simulink model "Taxi_park_hcs"  (R2022a)
settings: Solver=VariableStepAuto  StartTime=0.0  StopTime=10.0  RelTol=1e-3
settings Model: Creator=ayj  LastModifiedBy=ayj

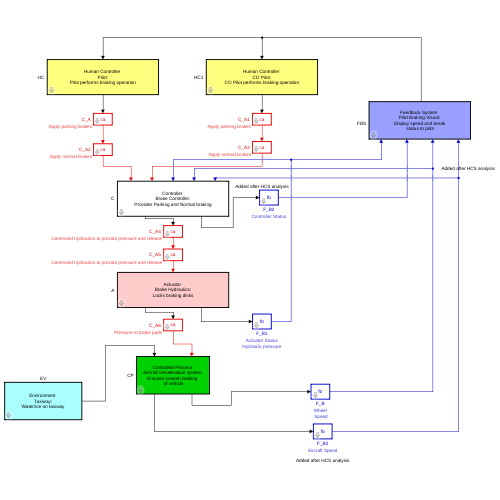
[thumbnail: Simulink's stored preview of the top-level diagram]
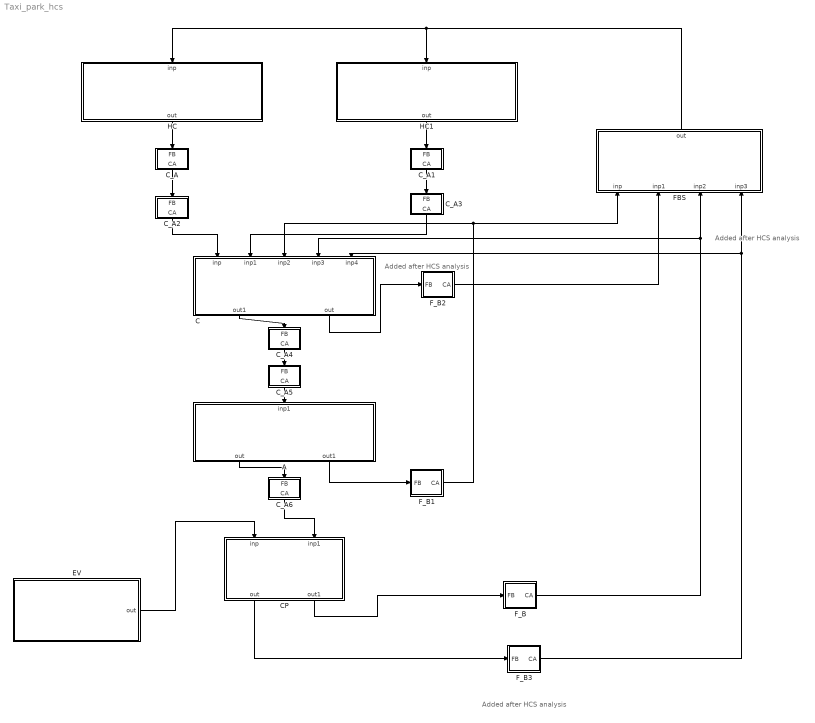
== system Taxi_park_hcs ==
  note: Added after HCS analysis
  note: Added after HCS analysis
  note: Added after HCS analysis
  " FBS" : Subsystem  TreatAsAtomicUnit=on  mask(feedback_system){NAMEFORBLOCK=Pilot Braking Visual, DES=Display speed and break\n status to pilot}
      mask prompts: NAMEFORBLOCK "Provide a name"; DES "Provide a description of feedback system"
      mask help: Say what this feedback system does
      mask init:
      | set_param(gcb,'LinkStatus', 'none');
      settings: RTWFcnNameOpts=Use subsystem name  RTWFileNameOpts=Use function name
      mask DialogControl Control2 Prompt: ADD Input
      mask DialogControl Control2 Callback:
      | h = add_block('simulink/Sources/In1', [gcb '/inp'], 'MakeNameUnique', 'on');
      | hg = add_block('simulink/Sinks/Terminator', [gcb '/term'], 'MakeNameUnique', 'on');
      | hname = get_param(h,'PortHandles');
      | hgname = get_param(hg,'PortHandles');
      | add_line(gcb, hname.Outport(1), hgname.Inport(1));
      mask DialogControl Control3 Prompt: ADD Output
      mask DialogControl Control3 Callback:
      | h = add_block('simulink/Sinks/Out1', [gcb '/out'], 'MakeNameUnique', 'on');
      | hg = add_block('simulink/Sources/Ground', [gcb '/gnd'], 'MakeNameUnique', 'on');
      | hname = get_param(h,'PortHandles');
      | hgname = get_param(hg,'PortHandles');
      | add_line(gcb, hgname.Outport(1), hname.Inport(1));
      mask DialogControl Control4 Prompt: REM Input
      mask DialogControl Control4 Callback:
      | a=find_system(gcb,'SearchDepth',2,'LookUnderMasks','all','BlockType','Inport');
      | if ~isempty(a)
      | b=get_param(a{1},'PortConnectivity');
      | delete_block(a{1});
      | delete_block(b.DstBlock);
      | delete_line(find_system(gcb, 'SearchDepth',2,'LookUnderMasks','all','FindAll', 'on', 'Type', 'line', 'Connected', 'off'))
      | end
      mask DialogControl Control5 Prompt: REM Output
      mask DialogControl Control5 Callback:
      | a=find_system(gcb,'SearchDepth',2,'LookUnderMasks','all','BlockType','Outport');
      | if ~isempty(a)
      | b=get_param(a{1},'PortConnectivity');
      | delete_block(a{1});
      | delete_block(b.SrcBlock);
      | delete_line(find_system(gcb, 'SearchDepth',2,'LookUnderMasks','all','FindAll', 'on', 'Type', 'line', 'Connected', 'off'))
      | end
      mask Display: disp(['Feedback System \n' NAMEFORBLOCK ':\n' DES])
  A : Subsystem  TreatAsAtomicUnit=on  mask(actuator){NAMEFORBLOCK=Brake Hydraulics, DES=Locks braking disks}
      mask prompts: NAMEFORBLOCK "Provide a name for Block"; DES "Provide a description of Responsibility"
      mask help: Say what this actuator does
      mask init:
      | set_param(gcb,'LinkStatus', 'none');
      settings: RTWFcnNameOpts=Use subsystem name  RTWFileNameOpts=Use function name
      mask DialogControl Control2 Prompt: ADD Input
      mask DialogControl Control2 Callback:
      | h = add_block('simulink/Sources/In1', [gcb '/inp'], 'MakeNameUnique', 'on');
      | hg = add_block('simulink/Sinks/Terminator', [gcb '/term'], 'MakeNameUnique', 'on');
      | hname = get_param(h,'PortHandles');
      | hgname = get_param(hg,'PortHandles');
      | add_line(gcb, hname.Outport(1), hgname.Inport(1));
      mask DialogControl Control3 Prompt: ADD Output
      mask DialogControl Control3 Callback:
      | h = add_block('simulink/Sinks/Out1', [gcb '/out'], 'MakeNameUnique', 'on');
      | hg = add_block('simulink/Sources/Ground', [gcb '/gnd'], 'MakeNameUnique', 'on');
      | hname = get_param(h,'PortHandles');
      | hgname = get_param(hg,'PortHandles');
      | add_line(gcb, hgname.Outport(1), hname.Inport(1));
      mask DialogControl Control4 Prompt: REM Input
      mask DialogControl Control4 Callback:
      | a=find_system(gcb,'SearchDepth',2,'LookUnderMasks','all','BlockType','Inport');
      | if ~isempty(a)
      | b=get_param(a{1},'PortConnectivity');
      | delete_block(a{1});
      | delete_block(b.DstBlock);
      | delete_line(find_system(gcb, 'SearchDepth',2,'LookUnderMasks','all','FindAll', 'on', 'Type', 'line', 'Connected', 'off'))
      | end
      mask DialogControl Control5 Prompt: REM Output
      mask DialogControl Control5 Callback:
      | a=find_system(gcb,'SearchDepth',2,'LookUnderMasks','all','BlockType','Outport');
      | if ~isempty(a)
      | b=get_param(a{1},'PortConnectivity');
      | delete_block(a{1});
      | delete_block(b.SrcBlock);
      | delete_line(find_system(gcb, 'SearchDepth',2,'LookUnderMasks','all','FindAll', 'on', 'Type', 'line', 'Connected', 'off'))
      | end
      mask Display: disp(['Actuator \n' NAMEFORBLOCK ':\n' DES])
  C : Subsystem  TreatAsAtomicUnit=on  mask(controller){NAMEFORBLOCK=Brake Controller, DES=Provides Parking and Normal braking}
      mask prompts: NAMEFORBLOCK "Provide a name for Block"; DES "Provide a description of Responsibility"
      mask help: Say what this controller does
      mask init:
      | set_param(gcb,'LinkStatus', 'none');
      settings: RTWFcnNameOpts=Use subsystem name  RTWFileNameOpts=Use function name
      mask DialogControl Control2 Prompt: ADD Input
      mask DialogControl Control2 Callback:
      | h = add_block('simulink/Sources/In1', [gcb '/inp'], 'MakeNameUnique', 'on');
      | hg = add_block('simulink/Sinks/Terminator', [gcb '/term'], 'MakeNameUnique', 'on');
      | hname = get_param(h,'PortHandles');
      | hgname = get_param(hg,'PortHandles');
      | add_line(gcb, hname.Outport(1), hgname.Inport(1));
      mask DialogControl Control3 Prompt: ADD Output
      mask DialogControl Control3 Callback:
      | h = add_block('simulink/Sinks/Out1', [gcb '/out'], 'MakeNameUnique', 'on');
      | hg = add_block('simulink/Sources/Ground', [gcb '/gnd'], 'MakeNameUnique', 'on');
      | hname = get_param(h,'PortHandles');
      | hgname = get_param(hg,'PortHandles');
      | add_line(gcb, hgname.Outport(1), hname.Inport(1));
      mask DialogControl Control4 Prompt: REM Input
      mask DialogControl Control4 Callback:
      | a=find_system(gcb,'SearchDepth',2,'LookUnderMasks','all','BlockType','Inport');
      | if ~isempty(a)
      | b=get_param(a{1},'PortConnectivity');
      | delete_block(a{1});
      | delete_block(b.DstBlock);
      | delete_line(find_system(gcb, 'SearchDepth',2,'LookUnderMasks','all','FindAll', 'on', 'Type', 'line', 'Connected', 'off'))
      | end
      mask DialogControl Control5 Prompt: REM Output
      mask DialogControl Control5 Callback:
      | a=find_system(gcb,'SearchDepth',2,'LookUnderMasks','all','BlockType','Outport');
      | if ~isempty(a)
      | b=get_param(a{1},'PortConnectivity');
      | delete_block(a{1});
      | delete_block(b.SrcBlock);
      | delete_line(find_system(gcb, 'SearchDepth',2,'LookUnderMasks','all','FindAll', 'on', 'Type', 'line', 'Connected', 'off'))
      | end
      mask Display: disp(['Controller \n' NAMEFORBLOCK ':\n' DES])
  CP : Subsystem  TreatAsAtomicUnit=on  mask(controlled_process){NAMEFORBLOCK=Aircraft Deceleration system, DES=Ensures smooth braking \n of vehicle}
      mask prompts: NAMEFORBLOCK "Provide a name for Block"; DES "Provide a description of Responsibility"
      mask help: Say what this controlled process does
      settings: RTWFcnNameOpts=Use subsystem name  RTWFileNameOpts=Use function name
      mask DialogControl Control2 Prompt: ADD Input
      mask DialogControl Control2 Callback:
      | set_param(gcb,'LinkStatus', 'none');
      | h = add_block('simulink/Sources/In1', [gcb '/inp'], 'MakeNameUnique', 'on');
      | hg = add_block('simulink/Sinks/Terminator', [gcb '/term'], 'MakeNameUnique', 'on');
      | hname = get_param(h,'PortHandles');
      | hgname = get_param(hg,'PortHandles');
      | add_line(gcb, hname.Outport(1), hgname.Inport(1));
      mask DialogControl Control3 Prompt: ADD Output
      mask DialogControl Control3 Callback:
      | set_param(gcb,'LinkStatus', 'none');
      | h = add_block('simulink/Sinks/Out1', [gcb '/out'], 'MakeNameUnique', 'on');
      | hg = add_block('simulink/Sources/Ground', [gcb '/gnd'], 'MakeNameUnique', 'on');
      | hname = get_param(h,'PortHandles');
      | hgname = get_param(hg,'PortHandles');
      | add_line(gcb, hgname.Outport(1), hname.Inport(1));
      mask DialogControl Control4 Prompt: REM Input
      mask DialogControl Control4 Callback:
      | set_param(gcb,'LinkStatus', 'none');
      | a=find_system(gcb,'SearchDepth',2,'LookUnderMasks','all','BlockType','Inport');
      | if ~isempty(a)
      | b=get_param(a{1},'PortConnectivity');
      | delete_block(a{1});
      | delete_block(b.DstBlock);
      | delete_line(find_system(gcb, 'SearchDepth',2,'LookUnderMasks','all','FindAll', 'on', 'Type', 'line', 'Connected', 'off'))
      | end
      mask DialogControl Control5 Prompt: REM Output
      mask DialogControl Control5 Callback:
      | set_param(gcb,'LinkStatus', 'none');
      | a=find_system(gcb,'SearchDepth',2,'LookUnderMasks','all','BlockType','Outport');
      | if ~isempty(a)
      | b=get_param(a{1},'PortConnectivity');
      | delete_block(a{1});
      | delete_block(b.SrcBlock);
      | delete_line(find_system(gcb, 'SearchDepth',2,'LookUnderMasks','all','FindAll', 'on', 'Type', 'line', 'Connected', 'off'))
      | end
      mask Display: disp(['Controlled Process \n' NAMEFORBLOCK ':\n' DES])
  C_A : Subsystem  TreatAsAtomicUnit=on  mask(control_action){DES=Apply parking brakes, UCA1=[#H5_1] Not providing at parking zone, UCA2=[#H4] Providing when taxing out, UCA3=[#H4] Providing early before aircraft has stopped, UCA4=}
      mask prompts: DES "Provide a description of Control Action"; UCA1 "Not providing causes hazard [link Hazard]"; UCA2 "Providing causes hazard [link Hazard]"; UCA3 "Too early, too late, out of order [link Hazard]"; UCA4 "Stopped too soon, applied too long [link Hazard]"
      mask help:
      | <Source> <Type> <Control Action> <Context> <Link to Hazards>
      | Source = System Above, Type = {provided, not provided ..], Control Action = command
      | from the description, Context = While/When .. Always link to a hazard
      mask init:
      | set_param(gcb,'LinkStatus', 'none');
      settings: AttributesFormatString=%<DES>  RTWFcnNameOpts=Use subsystem name  RTWFileNameOpts=Use function name
      mask Display: disp('ca')
  C_A1 : Subsystem  TreatAsAtomicUnit=on  mask(control_action){DES=Apply parking brakes, UCA1=[#H5_1] Not providing at parking zone, UCA2=[#H4] Providing when taxing out, UCA3=[#H4] Providing early before aircraft has stopped, UCA4=}
      mask prompts: DES "Provide a description of Control Action"; UCA1 "Not providing causes hazard [link Hazard]"; UCA2 "Providing causes hazard [link Hazard]"; UCA3 "Too early, too late, out of order [link Hazard]"; UCA4 "Stopped too soon, applied too long [link Hazard]"
      mask help:
      | <Source> <Type> <Control Action> <Context> <Link to Hazards>
      | Source = System Above, Type = {provided, not provided ..], Control Action = command
      | from the description, Context = While/When .. Always link to a hazard
      mask init:
      | set_param(gcb,'LinkStatus', 'none');
      settings: AttributesFormatString=%<DES>  RTWFcnNameOpts=Use subsystem name  RTWFileNameOpts=Use function name
      mask Display: disp('ca')
  C_A2 : Subsystem  TreatAsAtomicUnit=on  mask(control_action){DES=Apply normal brakes, UCA1=[#H5, #H6] Not applying brakes when instructed/needed, UCA2=[#H6] Providing without informing, UCA3=[#H4, #H7] erractic application of brakes, UCA4=[#H4, #H6] Release break before speed 0}
      mask prompts: DES "Provide a description of Control Action"; UCA1 "Not providing causes hazard [link Hazard]"; UCA2 "Providing causes hazard [link Hazard]"; UCA3 "Too early, too late, out of order [link Hazard]"; UCA4 "Stopped too soon, applied too long [link Hazard]"
      mask help:
      | <Source> <Type> <Control Action> <Context> <Link to Hazards>
      | Source = System Above, Type = {provided, not provided ..], Control Action = command
      | from the description, Context = While/When .. Always link to a hazard
      mask init:
      | set_param(gcb,'LinkStatus', 'none');
      settings: AttributesFormatString=%<DES>  RTWFcnNameOpts=Use subsystem name  RTWFileNameOpts=Use function name
      mask Display: disp('ca')
  C_A3 : Subsystem  TreatAsAtomicUnit=on  mask(control_action){DES=Apply normal brakes, UCA1=[#H5, #H6] Not applying brakes when instructed/needed, UCA2=[#H6] Providing without informing, UCA3=[#H4, #H7] erractic application of brakes, UCA4=[#H4, #H6] Release break before speed 0}
      mask prompts: DES "Provide a description of Control Action"; UCA1 "Not providing causes hazard [link Hazard]"; UCA2 "Providing causes hazard [link Hazard]"; UCA3 "Too early, too late, out of order [link Hazard]"; UCA4 "Stopped too soon, applied too long [link Hazard]"
      mask help:
      | <Source> <Type> <Control Action> <Context> <Link to Hazards>
      | Source = System Above, Type = {provided, not provided ..], Control Action = command
      | from the description, Context = While/When .. Always link to a hazard
      mask init:
      | set_param(gcb,'LinkStatus', 'none');
      settings: AttributesFormatString=%<DES>  RTWFcnNameOpts=Use subsystem name  RTWFileNameOpts=Use function name
      mask Display: disp('ca')
  C_A4 : Subsystem  TreatAsAtomicUnit=on  mask(control_action){DES=Command hydraulics to provide pressure and release, UCA1=[#H5, #H6] Not providing when demanded by pilot, UCA2=[#H5, #H6] Providing when pilot does not demand, UCA3=[#H5, #H6] Delayed brake action on command, UCA4=[#H5, #H6] Stopping brake pressure even under demand}
      mask prompts: DES "Provide a description of Control Action"; UCA1 "Not providing causes hazard [link Hazard]"; UCA2 "Providing causes hazard [link Hazard]"; UCA3 "Too early, too late, out of order [link Hazard]"; UCA4 "Stopped too soon, applied too long [link Hazard]"
      mask help:
      | <Source> <Type> <Control Action> <Context> <Link to Hazards>
      | Source = System Above, Type = {provided, not provided ..], Control Action = command
      | from the description, Context = While/When .. Always link to a hazard
      mask init:
      | set_param(gcb,'LinkStatus', 'none');
      settings: AttributesFormatString=%<DES>  RTWFcnNameOpts=Use subsystem name  RTWFileNameOpts=Use function name
      mask Display: disp('ca')
  C_A5 : Subsystem  TreatAsAtomicUnit=on  mask(control_action){DES=Command hydraulics to provide pressure and release, UCA1=, UCA2=[#H5, #H6] Providing unequal pressure to wheels, UCA3=[#H5, #H6] Either of the brakes are not in sync, UCA4=}
      mask prompts: DES "Provide a description of Control Action"; UCA1 "Not providing causes hazard [link Hazard]"; UCA2 "Providing causes hazard [link Hazard]"; UCA3 "Too early, too late, out of order [link Hazard]"; UCA4 "Stopped too soon, applied too long [link Hazard]"
      mask help:
      | <Source> <Type> <Control Action> <Context> <Link to Hazards>
      | Source = System Above, Type = {provided, not provided ..], Control Action = command
      | from the description, Context = While/When .. Always link to a hazard
      mask init:
      | set_param(gcb,'LinkStatus', 'none');
      settings: AttributesFormatString=%<DES>  RTWFcnNameOpts=Use subsystem name  RTWFileNameOpts=Use function name
      mask Display: disp('ca')
  C_A6 : Subsystem  TreatAsAtomicUnit=on  mask(control_action){DES=Pressure to brake pads, UCA1=[#H5, #H6] Not providing when demanded, UCA2=[#H5, #H6] Providing when not demanded, UCA3=[#H5, #H6] Providing pressure too late, UCA4=[#H5, #H6] Not releasing brake / Releasing too soon}
      mask prompts: DES "Provide a description of Control Action"; UCA1 "Not providing causes hazard [link Hazard]"; UCA2 "Providing causes hazard [link Hazard]"; UCA3 "Too early, too late, out of order [link Hazard]"; UCA4 "Stopped too soon, applied too long [link Hazard]"
      mask help:
      | <Source> <Type> <Control Action> <Context> <Link to Hazards>
      | Source = System Above, Type = {provided, not provided ..], Control Action = command
      | from the description, Context = While/When .. Always link to a hazard
      mask init:
      | set_param(gcb,'LinkStatus', 'none');
      settings: AttributesFormatString=%<DES>  RTWFcnNameOpts=Use subsystem name  RTWFileNameOpts=Use function name
      mask Display: disp('ca')
  EV : Subsystem  TreatAsAtomicUnit=on  mask(environment){NAMEFORBLOCK=Taxiway, DES=Water/ice on taxiway}
      mask prompts: NAMEFORBLOCK "Provide a name for Block"; DES "Provide a description of Interaction"
      mask help: Say how this environment interacts with the system
      mask init:
      | set_param(gcb,'LinkStatus', 'none');
      settings: RTWFcnNameOpts=Use subsystem name  RTWFileNameOpts=Use function name
      mask DialogControl Control2 Prompt: ADD Input
      mask DialogControl Control2 Callback:
      | h = add_block('simulink/Sources/In1', [gcb '/inp'], 'MakeNameUnique', 'on');
      | hg = add_block('simulink/Sinks/Terminator', [gcb '/term'], 'MakeNameUnique', 'on');
      | hname = get_param(h,'PortHandles');
      | hgname = get_param(hg,'PortHandles');
      | add_line(gcb, hname.Outport(1), hgname.Inport(1));
      mask DialogControl Control3 Prompt: ADD Output
      mask DialogControl Control3 Callback:
      | h = add_block('simulink/Sinks/Out1', [gcb '/out'], 'MakeNameUnique', 'on');
      | hg = add_block('simulink/Sources/Ground', [gcb '/gnd'], 'MakeNameUnique', 'on');
      | hname = get_param(h,'PortHandles');
      | hgname = get_param(hg,'PortHandles');
      | add_line(gcb, hgname.Outport(1), hname.Inport(1));
      mask DialogControl Control4 Prompt: REM Input
      mask DialogControl Control4 Callback:
      | a=find_system(gcb,'SearchDepth',2,'LookUnderMasks','all','BlockType','Inport');
      | if ~isempty(a)
      | b=get_param(a{1},'PortConnectivity');
      | delete_block(a{1});
      | delete_block(b.DstBlock);
      | delete_line(find_system(gcb, 'SearchDepth',2,'LookUnderMasks','all','FindAll', 'on', 'Type', 'line', 'Connected', 'off'))
      | end
      mask DialogControl Control5 Prompt: REM Output
      mask DialogControl Control5 Callback:
      | a=find_system(gcb,'SearchDepth',2,'LookUnderMasks','all','BlockType','Outport');
      | if ~isempty(a)
      | b=get_param(a{1},'PortConnectivity');
      | delete_block(a{1});
      | delete_block(b.SrcBlock);
      | delete_line(find_system(gcb, 'SearchDepth',2,'LookUnderMasks','all','FindAll', 'on', 'Type', 'line', 'Connected', 'off'))
      | end
      mask Display: disp(['Environment \n' NAMEFORBLOCK ':\n' DES])
  F_B : Subsystem  TreatAsAtomicUnit=on  mask(feedback){DES=Wheel\n Speed}
      mask prompts: DES "Provide a description"
      mask help: Say what this feeds back from the system
      mask init:
      | set_param(gcb,'LinkStatus', 'none');
      settings: AttributesFormatString=%<DES>  RTWFcnNameOpts=Use subsystem name  RTWFileNameOpts=Use function name
      mask Display: disp('fb')
  F_B1 : Subsystem  TreatAsAtomicUnit=on  mask(feedback){DES=Actuator Status\nHydraulic pressure}
      mask prompts: DES "Provide a description"
      mask help: Say what this feeds back from the system
      mask init:
      | set_param(gcb,'LinkStatus', 'none');
      settings: AttributesFormatString=%<DES>  RTWFcnNameOpts=Use subsystem name  RTWFileNameOpts=Use function name
      mask Display: disp('fb')
  F_B2 : Subsystem  TreatAsAtomicUnit=on  mask(feedback){DES=Controller Status}
      mask prompts: DES "Provide a description"
      mask help: Say what this feeds back from the system
      mask init:
      | set_param(gcb,'LinkStatus', 'none');
      settings: AttributesFormatString=%<DES>  RTWFcnNameOpts=Use subsystem name  RTWFileNameOpts=Use function name
      mask Display: disp('fb')
  F_B3 : Subsystem  TreatAsAtomicUnit=on  mask(feedback){DES=Aircraft Speed}
      mask prompts: DES "Provide a description"
      mask help: Say what this feeds back from the system
      mask init:
      | set_param(gcb,'LinkStatus', 'none');
      settings: AttributesFormatString=%<DES>  RTWFcnNameOpts=Use subsystem name  RTWFileNameOpts=Use function name
      mask Display: disp('fb')
  HC : Subsystem  TreatAsAtomicUnit=on  mask(human_controller){NAMEFORBLOCK=Pilot, DES=Pilot performs braking operation}
      mask prompts: NAMEFORBLOCK "Provide a name for Block"; DES "Provide a description of Responsibility"
      mask help: Say what this human controller does
      mask init:
      | set_param(gcb,'LinkStatus','none')
      settings: RTWFcnNameOpts=Use subsystem name  RTWFileNameOpts=Use function name
      mask DialogControl Control2 Prompt: ADD Input
      mask DialogControl Control2 Callback:
      | h = add_block('simulink/Sources/In1', [gcb '/inp'], 'MakeNameUnique', 'on');
      | hg = add_block('simulink/Sinks/Terminator', [gcb '/term'], 'MakeNameUnique', 'on');
      | hname = get_param(h,'PortHandles');
      | hgname = get_param(hg,'PortHandles');
      | add_line(gcb, hname.Outport(1), hgname.Inport(1));
      mask DialogControl Control3 Prompt: ADD Output
      mask DialogControl Control3 Callback:
      | h = add_block('simulink/Sinks/Out1', [gcb '/out'], 'MakeNameUnique', 'on');
      | hg = add_block('simulink/Sources/Ground', [gcb '/gnd'], 'MakeNameUnique', 'on');
      | hname = get_param(h,'PortHandles');
      | hgname = get_param(hg,'PortHandles');
      | add_line(gcb, hgname.Outport(1), hname.Inport(1));
      mask DialogControl Control4 Prompt: REM Input
      mask DialogControl Control4 Callback:
      | a=find_system(gcb,'SearchDepth',2,'LookUnderMasks','all','BlockType','Inport');
      | if ~isempty(a)
      | b=get_param(a{1},'PortConnectivity');
      | delete_block(a{1});
      | delete_block(b.DstBlock);
      | delete_line(find_system(gcb, 'SearchDepth',2,'LookUnderMasks','all','FindAll', 'on', 'Type', 'line', 'Connected', 'off'))
      | end
      mask DialogControl Control5 Prompt: REM Output
      mask DialogControl Control5 Callback:
      | a=find_system(gcb,'SearchDepth',2,'LookUnderMasks','all','BlockType','Outport');
      | if ~isempty(a)
      | b=get_param(a{1},'PortConnectivity');
      | delete_block(a{1});
      | delete_block(b.SrcBlock);
      | delete_line(find_system(gcb, 'SearchDepth',2,'LookUnderMasks','all','FindAll', 'on', 'Type', 'line', 'Connected', 'off'))
      | end
      mask Display: disp(['Human Controller \n' NAMEFORBLOCK ':\n' DES])
  HC1 : Subsystem  TreatAsAtomicUnit=on  mask(human_controller){NAMEFORBLOCK=CO Pilot, DES=CO Pilot performs braking operation}
      mask prompts: NAMEFORBLOCK "Provide a name for Block"; DES "Provide a description of Responsibility"
      mask help: Say what this human controller does
      mask init:
      | set_param(gcb,'LinkStatus','none')
      settings: RTWFcnNameOpts=Use subsystem name  RTWFileNameOpts=Use function name
      mask DialogControl Control2 Prompt: ADD Input
      mask DialogControl Control2 Callback:
      | h = add_block('simulink/Sources/In1', [gcb '/inp'], 'MakeNameUnique', 'on');
      | hg = add_block('simulink/Sinks/Terminator', [gcb '/term'], 'MakeNameUnique', 'on');
      | hname = get_param(h,'PortHandles');
      | hgname = get_param(hg,'PortHandles');
      | add_line(gcb, hname.Outport(1), hgname.Inport(1));
      mask DialogControl Control3 Prompt: ADD Output
      mask DialogControl Control3 Callback:
      | h = add_block('simulink/Sinks/Out1', [gcb '/out'], 'MakeNameUnique', 'on');
      | hg = add_block('simulink/Sources/Ground', [gcb '/gnd'], 'MakeNameUnique', 'on');
      | hname = get_param(h,'PortHandles');
      | hgname = get_param(hg,'PortHandles');
      | add_line(gcb, hgname.Outport(1), hname.Inport(1));
      mask DialogControl Control4 Prompt: REM Input
      mask DialogControl Control4 Callback:
      | a=find_system(gcb,'SearchDepth',2,'LookUnderMasks','all','BlockType','Inport');
      | if ~isempty(a)
      | b=get_param(a{1},'PortConnectivity');
      | delete_block(a{1});
      | delete_block(b.DstBlock);
      | delete_line(find_system(gcb, 'SearchDepth',2,'LookUnderMasks','all','FindAll', 'on', 'Type', 'line', 'Connected', 'off'))
      | end
      mask DialogControl Control5 Prompt: REM Output
      mask DialogControl Control5 Callback:
      | a=find_system(gcb,'SearchDepth',2,'LookUnderMasks','all','BlockType','Outport');
      | if ~isempty(a)
      | b=get_param(a{1},'PortConnectivity');
      | delete_block(a{1});
      | delete_block(b.SrcBlock);
      | delete_line(find_system(gcb, 'SearchDepth',2,'LookUnderMasks','all','FindAll', 'on', 'Type', 'line', 'Connected', 'off'))
      | end
      mask Display: disp(['Human Controller \n' NAMEFORBLOCK ':\n' DES])
  wires:
  HC/1(out) -> C_A/1(FB)
  C_A/1(CA) -> C_A2/1(FB)
  C_A1/1(CA) -> C_A3/1(FB)
  HC1/1(out) -> C_A1/1(FB)
  C_A2/1(CA) -> C/1(inp)
  C_A3/1(CA) -> C/2(inp1)
  C/1(out1) -> C_A4/1(FB)
  C_A4/1(CA) -> C_A5/1(FB)
  C_A5/1(CA) -> A/1(inp1)
  A/1(out) -> C_A6/1(FB)
  C_A6/1(CA) -> CP/2(inp1)
  " FBS"/1(out) -> HC1/1(inp), HC/1(inp)
  CP/2(out1) -> F_B/1(FB)
  F_B/1(CA) -> " FBS"/3(inp2), C/4(inp3)
  A/2(out1) -> F_B1/1(FB)
  F_B1/1(CA) -> " FBS"/1(inp), C/3(inp2)
  EV/1(out) -> CP/1(inp)
  C/2(out) -> F_B2/1(FB)
  F_B2/1(CA) -> " FBS"/2(inp1)
  CP/1(out) -> F_B3/1(FB)
  F_B3/1(CA) -> C/5(inp4), " FBS"/4(inp3)

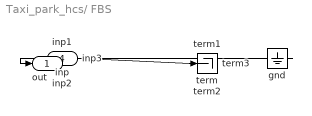
== system Taxi_park_hcs/ FBS ==
  inp : Inport
  inp1 : Inport  Port=2
  inp2 : Inport  Port=3
  inp3 : Inport  Port=4
  gnd : Ground
  term{,1..3} (4 alike) : Terminator
  out : Outport
  wires:
  inp/1 -> term/1
  gnd/1 -> out/1
  inp1/1 -> term1/1
  inp2/1 -> term2/1
  inp3/1 -> term3/1

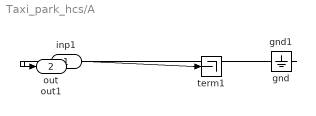
== system Taxi_park_hcs/A ==
  inp1 : Inport
  gnd : Ground
  gnd1 : Ground
  term1 : Terminator
  out : Outport
  out1 : Outport  Port=2
  wires:
  gnd/1 -> out/1
  inp1/1 -> term1/1
  gnd1/1 -> out1/1

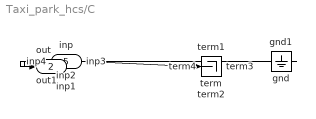
== system Taxi_park_hcs/C ==
  inp : Inport
  inp1 : Inport  Port=2
  inp2 : Inport  Port=3
  inp3 : Inport  Port=4
  inp4 : Inport  Port=5
  gnd : Ground
  gnd1 : Ground
  term{,1..4} (5 alike) : Terminator
  out1 : Outport
  out : Outport  Port=2
  wires:
  inp/1 -> term/1
  inp1/1 -> term1/1
  gnd1/1 -> out1/1
  inp2/1 -> term2/1
  gnd/1 -> out/1
  inp3/1 -> term3/1
  inp4/1 -> term4/1

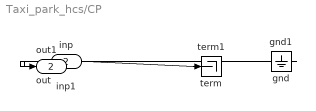
== system Taxi_park_hcs/CP ==
  inp : Inport
  inp1 : Inport  Port=2
  gnd : Ground
  gnd1 : Ground
  term : Terminator
  term1 : Terminator
  out : Outport
  out1 : Outport  Port=2
  wires:
  gnd/1 -> out/1
  inp/1 -> term/1
  inp1/1 -> term1/1
  gnd1/1 -> out1/1

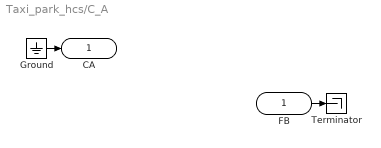
== system Taxi_park_hcs/C_A ==
  FB : Inport
      mask Display:
      | plot([0 60-10],[0 0]);
      | plot([0 0],[0 16]);
      | plot([0 60-10],[16 16]);
      | plot([60-10 60],[16 8]);
      | plot([60-10 60],[0 8]);
  Ground : Ground
  Terminator : Terminator
  CA : Outport
      mask Display:
      | plot([10 65],[0 0]);
      | plot([65-1 65-1],[0 16]);
      | plot([10 65],[16 16]);
      | plot([0 10],[8 16]);
      | plot([0 10],[8 0]);
  wires:
  Ground/1 -> CA/1
  FB/1 -> Terminator/1

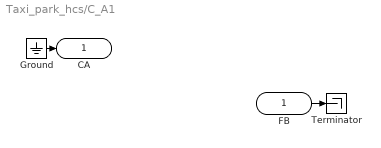
== system Taxi_park_hcs/C_A1 ==
  FB : Inport
      mask Display:
      | plot([0 60-10],[0 0]);
      | plot([0 0],[0 16]);
      | plot([0 60-10],[16 16]);
      | plot([60-10 60],[16 8]);
      | plot([60-10 60],[0 8]);
  Ground : Ground
  Terminator : Terminator
  CA : Outport
      mask Display:
      | plot([10 65],[0 0]);
      | plot([65-1 65-1],[0 16]);
      | plot([10 65],[16 16]);
      | plot([0 10],[8 16]);
      | plot([0 10],[8 0]);
  wires:
  FB/1 -> Terminator/1
  Ground/1 -> CA/1

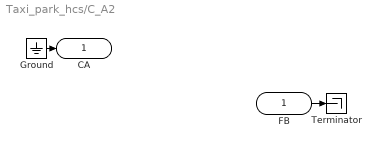
== system Taxi_park_hcs/C_A2 ==
  FB : Inport
      mask Display:
      | plot([0 60-10],[0 0]);
      | plot([0 0],[0 16]);
      | plot([0 60-10],[16 16]);
      | plot([60-10 60],[16 8]);
      | plot([60-10 60],[0 8]);
  Ground : Ground
  Terminator : Terminator
  CA : Outport
      mask Display:
      | plot([10 65],[0 0]);
      | plot([65-1 65-1],[0 16]);
      | plot([10 65],[16 16]);
      | plot([0 10],[8 16]);
      | plot([0 10],[8 0]);
  wires:
  Ground/1 -> CA/1
  FB/1 -> Terminator/1

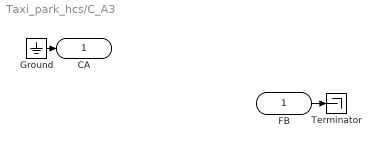
== system Taxi_park_hcs/C_A3 ==
  FB : Inport
      mask Display:
      | plot([0 60-10],[0 0]);
      | plot([0 0],[0 16]);
      | plot([0 60-10],[16 16]);
      | plot([60-10 60],[16 8]);
      | plot([60-10 60],[0 8]);
  Ground : Ground
  Terminator : Terminator
  CA : Outport
      mask Display:
      | plot([10 65],[0 0]);
      | plot([65-1 65-1],[0 16]);
      | plot([10 65],[16 16]);
      | plot([0 10],[8 16]);
      | plot([0 10],[8 0]);
  wires:
  FB/1 -> Terminator/1
  Ground/1 -> CA/1

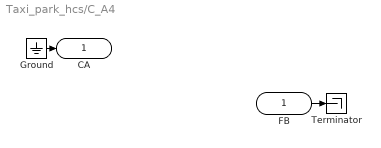
== system Taxi_park_hcs/C_A4 ==
  FB : Inport
      mask Display:
      | plot([0 60-10],[0 0]);
      | plot([0 0],[0 16]);
      | plot([0 60-10],[16 16]);
      | plot([60-10 60],[16 8]);
      | plot([60-10 60],[0 8]);
  Ground : Ground
  Terminator : Terminator
  CA : Outport
      mask Display:
      | plot([10 65],[0 0]);
      | plot([65-1 65-1],[0 16]);
      | plot([10 65],[16 16]);
      | plot([0 10],[8 16]);
      | plot([0 10],[8 0]);
  wires:
  Ground/1 -> CA/1
  FB/1 -> Terminator/1

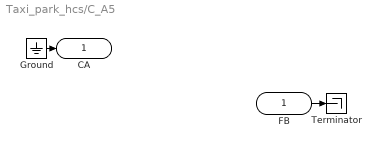
== system Taxi_park_hcs/C_A5 ==
  FB : Inport
      mask Display:
      | plot([0 60-10],[0 0]);
      | plot([0 0],[0 16]);
      | plot([0 60-10],[16 16]);
      | plot([60-10 60],[16 8]);
      | plot([60-10 60],[0 8]);
  Ground : Ground
  Terminator : Terminator
  CA : Outport
      mask Display:
      | plot([10 65],[0 0]);
      | plot([65-1 65-1],[0 16]);
      | plot([10 65],[16 16]);
      | plot([0 10],[8 16]);
      | plot([0 10],[8 0]);
  wires:
  FB/1 -> Terminator/1
  Ground/1 -> CA/1

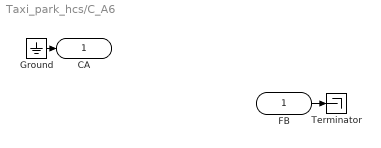
== system Taxi_park_hcs/C_A6 ==
  FB : Inport
      mask Display:
      | plot([0 60-10],[0 0]);
      | plot([0 0],[0 16]);
      | plot([0 60-10],[16 16]);
      | plot([60-10 60],[16 8]);
      | plot([60-10 60],[0 8]);
  Ground : Ground
  Terminator : Terminator
  CA : Outport
      mask Display:
      | plot([10 65],[0 0]);
      | plot([65-1 65-1],[0 16]);
      | plot([10 65],[16 16]);
      | plot([0 10],[8 16]);
      | plot([0 10],[8 0]);
  wires:
  Ground/1 -> CA/1
  FB/1 -> Terminator/1

== system Taxi_park_hcs/EV ==
  gnd : Ground
  out : Outport
  wires:
  gnd/1 -> out/1

== system Taxi_park_hcs/F_B ==
  FB : Inport
      mask Display:
      | plot([0 60-10],[0 0]);
      | plot([0 0],[0 16]);
      | plot([0 60-10],[16 16]);
      | plot([60-10 60],[16 8]);
      | plot([60-10 60],[0 8]);
  Ground : Ground
  Terminator : Terminator
  CA : Outport
      mask Display:
      | plot([10 65],[0 0]);
      | plot([65-1 65-1],[0 16]);
      | plot([10 65],[16 16]);
      | plot([0 10],[8 16]);
      | plot([0 10],[8 0]);
  wires:
  FB/1 -> Terminator/1
  Ground/1 -> CA/1

== system Taxi_park_hcs/F_B1 ==
  FB : Inport
      mask Display:
      | plot([0 60-10],[0 0]);
      | plot([0 0],[0 16]);
      | plot([0 60-10],[16 16]);
      | plot([60-10 60],[16 8]);
      | plot([60-10 60],[0 8]);
  Ground : Ground
  Terminator : Terminator
  CA : Outport
      mask Display:
      | plot([10 65],[0 0]);
      | plot([65-1 65-1],[0 16]);
      | plot([10 65],[16 16]);
      | plot([0 10],[8 16]);
      | plot([0 10],[8 0]);
  wires:
  Ground/1 -> CA/1
  FB/1 -> Terminator/1

== system Taxi_park_hcs/F_B2 ==
  FB : Inport
      mask Display:
      | plot([0 60-10],[0 0]);
      | plot([0 0],[0 16]);
      | plot([0 60-10],[16 16]);
      | plot([60-10 60],[16 8]);
      | plot([60-10 60],[0 8]);
  Ground : Ground
  Terminator : Terminator
  CA : Outport
      mask Display:
      | plot([10 65],[0 0]);
      | plot([65-1 65-1],[0 16]);
      | plot([10 65],[16 16]);
      | plot([0 10],[8 16]);
      | plot([0 10],[8 0]);
  wires:
  FB/1 -> Terminator/1
  Ground/1 -> CA/1

== system Taxi_park_hcs/F_B3 ==
  FB : Inport
      mask Display:
      | plot([0 60-10],[0 0]);
      | plot([0 0],[0 16]);
      | plot([0 60-10],[16 16]);
      | plot([60-10 60],[16 8]);
      | plot([60-10 60],[0 8]);
  Ground : Ground
  Terminator : Terminator
  CA : Outport
      mask Display:
      | plot([10 65],[0 0]);
      | plot([65-1 65-1],[0 16]);
      | plot([10 65],[16 16]);
      | plot([0 10],[8 16]);
      | plot([0 10],[8 0]);
  wires:
  Ground/1 -> CA/1
  FB/1 -> Terminator/1

== system Taxi_park_hcs/HC ==
  inp : Inport
  gnd : Ground
  term : Terminator
  out : Outport
  wires:
  gnd/1 -> out/1
  inp/1 -> term/1

== system Taxi_park_hcs/HC1 ==
  inp : Inport
  gnd : Ground
  term : Terminator
  out : Outport
  wires:
  inp/1 -> term/1
  gnd/1 -> out/1
